simulink model "test"  (Simulink 6.0)
settings: Solver=ode45  StartTime=0.0  StopTime=3  RelTol=1e-3
settings Model: LastModifiedBy=Jayantha

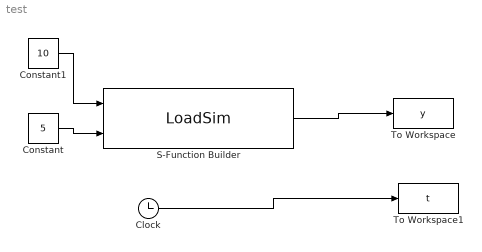
== system test ==
  Clock : Clock
      settings: Decimation=10
  Constant : Constant  Value=5
  Constant1 : Constant  Value=10
  S-Function Builder : S-Function  InitFcn=try, set_param(gcb,'FunctionName','LoadSim'), end,  FunctionName=LoadSim  SFunctionModules=LoadSim_wrapper  WizardData=DataTag0  mask(S-Function Builder){}
      mask init:
      | val = [[.9  0.75 0.75 1 1 .9 .9 1]',[1 1 0.75 0.75 .9 .9 1 .9]'];try , sys = get_param(gcb,'SfunBuilderFcnName');if isempty(sys), sys = get_param(gcb,'FunctionName'); end,catch, sys = get_param(gcb,'FunctionName'); end
      settings: CopyFcn=set_param(gcbh,'LinkStatus','none')  PreSaveFcn=try, set_param(gcb,'FunctionName','LoadSim'), end  OpenFcn=sfunctionwizard(gcbh)
      mask Display: plot(val(:,1),val(:,2)),disp(sys)port_label('input',1,'u0')port_label('input',2,'u1')port_label('output',1,'y0')
  To Workspace : ToWorkspace  VariableName=y  SampleTime=-1  SaveFormat=Array
  To Workspace1 : ToWorkspace  VariableName=t  SampleTime=-1  SaveFormat=Array
  wires:
  Constant/1 -> S-Function Builder/2
  Constant1/1 -> S-Function Builder/1
  S-Function Builder/1 -> To Workspace/1
  Clock/1 -> To Workspace1/1
